simulink subsystem "NoSuspension"  (R2024b)
settings: Solver=VariableStepAuto  StartTime=0.0  StopTime=10.0  RelTol=1e-3
settings Model: ModifiedByFormat=The MathWorks, Inc.  Creator=The MathWorks, Inc.  LastModifiedBy=The MathWorks, Inc.
settings OptimizationCC: ReuseModelBlockBuffer=off
settings DebuggingCC: SubsystemReferenceDiagnosticForUnitTest=warning
settings RTWCC: GPUComputeCapability=3.5

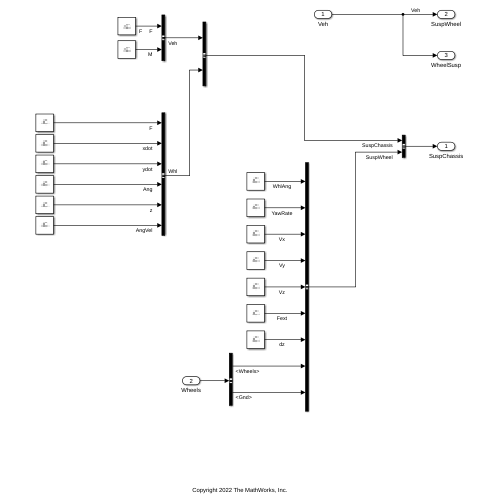
[thumbnail: Simulink's stored preview of the top-level diagram]
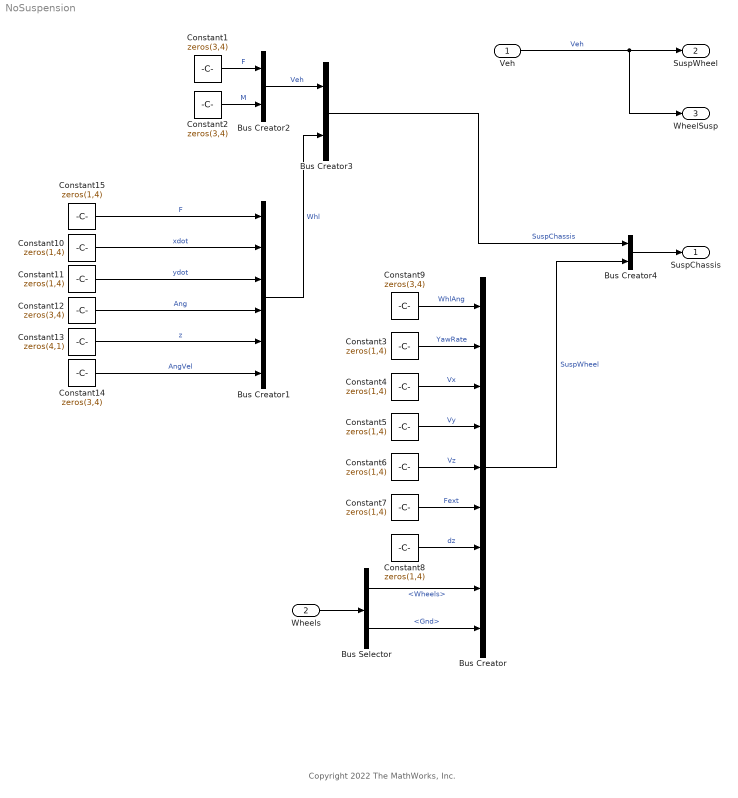
== system NoSuspension ==
  note: Copyright 2022 The MathWorks, Inc.
  Veh : Inport
  Wheels : Inport  Port=2
  Bus Creator : BusCreator  Inputs=9
  Bus Creator1 : BusCreator  Inputs=6
  Bus Creator2 : BusCreator  Inputs=2
  Bus Creator3 : BusCreator  Inputs=2
  Bus Creator4 : BusCreator  Inputs=2
  Bus Selector : BusSelector  OutputSignals=Wheels,Gnd
  Constant{1..2,9,12,14} (5 alike) : Constant  Value=zeros(3,4)  SampleTime=-1
  Constant{3..8,10..11,15} (9 alike) : Constant  Value=zeros(1,4)  SampleTime=-1
  Constant13 : Constant  Value=zeros(4,1)  SampleTime=-1
  SuspChassis : Outport
  SuspWheel : Outport  Port=2
  WheelSusp : Outport  Port=3
  wires:
  Constant15/1 -> Bus Creator1/1  "F"
  Constant11/1 -> Bus Creator1/3  "ydot"
  Constant12/1 -> Bus Creator1/4  "Ang"
  Bus Creator1/1 -> Bus Creator3/2  "Whl"
  Constant10/1 -> Bus Creator1/2  "xdot"
  Constant13/1 -> Bus Creator1/5  "z"
  Constant14/1 -> Bus Creator1/6  "AngVel"
  Bus Creator/1 -> Bus Creator4/2  "SuspWheel"
  Bus Creator3/1 -> Bus Creator4/1  "SuspChassis"
  Veh/1 -> SuspWheel/1, WheelSusp/1  "Veh"
  Bus Creator4/1 -> SuspChassis/1
  Bus Creator2/1 -> Bus Creator3/1  "Veh"
  Constant1/1 -> Bus Creator2/1  "F"
  Constant2/1 -> Bus Creator2/2  "M"
  Constant8/1 -> Bus Creator/7  "dz"
  Constant9/1 -> Bus Creator/1  "WhlAng"
  Constant4/1 -> Bus Creator/3  "Vx"
  Constant7/1 -> Bus Creator/6  "Fext"
  Constant6/1 -> Bus Creator/5  "Vz"
  Constant3/1 -> Bus Creator/2  "YawRate"
  Constant5/1 -> Bus Creator/4  "Vy"
  Wheels/1 -> Bus Selector/1
  Bus Selector/1 -> Bus Creator/8  "<Wheels>"
  Bus Selector/2 -> Bus Creator/9  "<Gnd>"
